simulink model "highspeed_iobuf_ex"  (Simulink 7.1)
settings: Solver=ode45  StartTime=0.0  StopTime=1000  RelTol=1e-3
libraries: xbsIndex_r4 x32, xbsCopyrightNotice_r4 x1
settings Model: Creator=alexc  LastModifiedBy=juttu
settings DataIOCC: SignalLoggingName=sigsOut
settings DebuggingCC: SaveWithParameterizedLinksMsg=none  SignalResolutionControl=TryResolveAllWithWarning  SolverPrmCheckMsg=none  MultiTaskDSMMsg=warning  MultiTaskCondExecSysMsg=none  StrictBusMsg=None
settings HardwareCC: TargetUnknown=on
settings RTWCC: IncludeERTFirstTime=on
settings GRTTargetCC: TargetFcnLib=ansi_tfl_tmw.mat

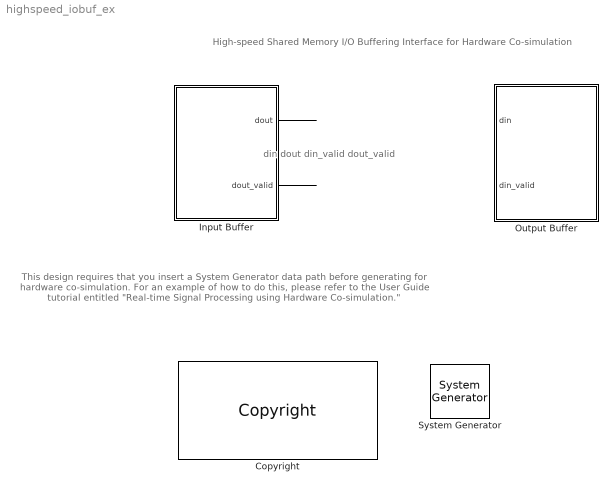
== system highspeed_iobuf_ex ==
  note: din                     dout
      |
      |
      |
      |
      | din_valid   dout_valid
  note: High-speed Shared Memory I/O Buffering Interface
      | for Hardware Co-simulation
  note: This design requires that you insert a System Generator
      | data path before generating for hardware co-simulation.
      | For an example of how to do this, please refer to the User
      | Guide tutorial entitled "Real-time Signal Processing using
      | Hardware Co-simulation."
  " System Generator" : xbsIndex_r4/ System Generator  Tag=genX  SystemSampleTime=-1  xilinxfamily=virtex4  part=xc4vsx35  speed=-10  package=ff668  synthesis_tool=XST  clock_wrapper=Clock Enables  directory=./netlist  testbench=off  simulink_period=1  sysclk_period=25  dcm_input_clock_period=100  incr_netlist=off  trim_vbits=Everywhere in SubSystem  dbl_ovrd=According to Block Masks  core_generation=According to Block Masks  run_coregen=off  deprecated_control=off  eval_field=0  block_type=sysgen
      settings: block_version=11.1
  Copyright : xbsCopyrightNotice_r4/Copyright  copyrighttext="Copyright (c) 2009  by  Xilinx, Inc. All rights reserved.<br><br>This file contains proprietary, confidential information of Xilinx, Inc., is distributed under licensefrom Xilinx, Inc., and may be used, copied and/or disclosed only pursuant to the terms of a valid licenseagreement with Xilinx, Inc. Xilinx hereby grants you a license to use this file solely for design,simulation, implementation and creation of design files limited to Xilinx devices or technologies. Use with non-Xilinx devices or technologies is expressly prohibited and immediately terminates your license unless covered by a separate agreement.<br><br>Xilinx is providing this design, code, or information \"as-is\" solely for use in developing programs and solutions for Xilinx devices, with no obligation on the part of Xilinx to provide support. By providingthis design, code, or information as one possible implementation of this feature, application or standard,Xilinx is making no representation that this implementation is free from any claims of infringement. Youare responsible for obtaining any rights you may require for your implementation. Xilinx expressly disclaimsany warranty whatsoever with respect to the adequacy of the implementation, including but not limited to anywarranties or representations that this implementation is free from claims of infringement, implied warrantiesof merchantability or fitness for a particular purpose.<br><br>Xilinx products are not intended for use in life support appliances, devices, or systems. Use in such applications is expressly prohibited.<br><br>Any modifications that are made to the Source Code are done at the user's sole risk and will be unsupported.<br><br>This copyright and support notice must be retained as part of this text at all times. (c) Copyright 1995-2009 Xilinx, Inc. All rights reserved."  block_type=copyright
      settings: block_version=11.1
  Input Buffer : Subsystem  mask{smName='Foo', smDepth=128*128, smWidth=8}
      mask prompts: smName "Shared Memory Name"; smDepth "Shared Memory Depth"; smWidth "Shared Memory Width"
  Output Buffer : Subsystem  mask{smName='Bar', smDepth=128*128}
      mask prompts: smName "Shared Memory Name"; smDepth "Shared Memory Depth"
  wires:
  Input Buffer/1(dout) -> ?
  Input Buffer/2(dout_valid) -> ?
  ? -> Output Buffer/1(din)
  ? -> Output Buffer/2(din_valid)

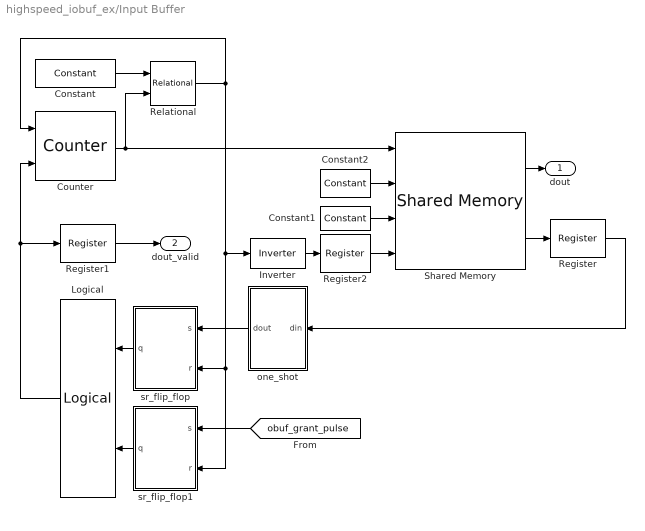
== system highspeed_iobuf_ex/Input Buffer ==
  Constant : xbsIndex_r4/Constant  arith_type=Unsigned  const=smDepth-1  n_bits=ceil(log2(smDepth))  bin_pt=0  explicit_period=on  period=1  equ=P=C  opselect=C  inp2=PCIN>>17  opr=+  inp1=P  carry=CIN  dbl_ovrd=off  block_type=constant
      settings: block_version=VER_STRING_GOES_HERE
  Constant1 : xbsIndex_r4/Constant  arith_type=Boolean  const=0  n_bits=1  bin_pt=0  explicit_period=off  period=1  equ=P=C  opselect=C  inp2=PCIN>>17  opr=+  inp1=P  carry=CIN  dbl_ovrd=off  block_type=constant
      settings: block_version=VER_STRING_GOES_HERE
  Constant2 : xbsIndex_r4/Constant  arith_type=Unsigned  const=0  n_bits=smWidth  bin_pt=0  explicit_period=off  period=1  equ=P=C  opselect=C  inp2=PCIN>>17  opr=+  inp1=P  carry=CIN  dbl_ovrd=off  block_type=constant
      settings: block_version=VER_STRING_GOES_HERE
  Counter : xbsIndex_r4/Counter  cnt_type=Free Running  cnt_to=Inf  operation=Up  start_count=0  cnt_by_val=1  arith_type=Unsigned  n_bits=ceil(log2(smDepth))  bin_pt=0  load_pin=off  rst=on  en=on  dbl_ovrd=off  explicit_period=on  period=1  use_behavioral_HDL=off  use_rpm=off  block_type=counter
      settings: infoedit="Configurable up, down and up/down counter.<P><P>Hardware notes: Free running counters are the least expensive in hardware.  A count limited counter is implemented by combining a counter with a comparator."  xl_area=[0, 0, 0, 0, 0, 0, 0]  block_version=VER_STRING_GOES_HERE
  Inverter : xbsIndex_r4/Inverter  en=off  latency=0  dbl_ovrd=off  block_type=inv
      settings: xl_area=[0, 0, 0, 0, 0, 0, 0]  block_version=VER_STRING_GOES_HERE
  Logical : xbsIndex_r4/Logical  Orientation=left  logical_function=AND  inputs=2  en=off  latency=0  precision=Full  arith_type=Unsigned  n_bits=8  bin_pt=2  align_bp=on  dbl_ovrd=off  block_type=logical
      settings: xl_area=[0, 0, 0, 0, 0, 0, 0]  block_version=VER_STRING_GOES_HERE
  Register : xbsIndex_r4/Register  init=0  rst=off  en=off  dbl_ovrd=off  block_type=register
      settings: xl_area=[0, 0, 0, 0, 0, 0, 0]  block_version=VER_STRING_GOES_HERE
  Register1 : xbsIndex_r4/Register  init=0  rst=off  en=off  dbl_ovrd=off  block_type=register
      settings: xl_area=[0, 0, 0, 0, 0, 0, 0]  block_version=VER_STRING_GOES_HERE
  Register2 : xbsIndex_r4/Register  init=0  rst=off  en=off  dbl_ovrd=off  block_type=register
      settings: xl_area=[0, 0, 0, 0, 0, 0, 0]  block_version=VER_STRING_GOES_HERE
  Relational : xbsIndex_r4/Relational  mode=a=b  en=off  latency=0  dbl_ovrd=off  block_type=relational
      settings: xl_area=[0, 0, 0, 0, 0, 0, 0]  block_version=VER_STRING_GOES_HERE
  Shared Memory : xbsIndex_r4/Shared Memory  shared_memory_name=smName  depth=smDepth  ownership=Locally Owned and Initialized  initVector=0:255  mutex=Lockable  mode=Read and Write  write_mode=Read After Write  time_out=0  explicit_data_type=off  arith_type=Unsigned  n_bits=0  bin_pt=0  implementation=Block RAM  use_rpm=off  block_type=shmem
      settings: AttributesFormatString=<< %<shared_memory_name> >>  xl_area=[0, 0, 0, 0, 0, 0, 0]  block_version=VER_STRING_GOES_HERE
  one_shot : Subsystem  Orientation=left
  sr_flip_flop : Subsystem  Orientation=left
  sr_flip_flop1 : Subsystem  Orientation=left
  dout : Outport  OutDataType=sfix(16)  OutScaling=2^0
  dout_valid : Outport  Port=2  OutDataType=sfix(16)  OutScaling=2^0
  wires:
  Shared Memory/2 -> Register/1
  Counter/1 -> Shared Memory/1, Relational/2
  Constant/1 -> Relational/1
  Relational/1 -> Inverter/1, sr_flip_flop/2(r), sr_flip_flop1/2(r), Counter/1
  Inverter/1 -> Register2/1
  Register2/1 -> Shared Memory/4
  Constant1/1 -> Shared Memory/3
  Constant2/1 -> Shared Memory/2
  [obuf_grant_pulse] -> sr_flip_flop1/1(s)
  one_shot/1(dout) -> sr_flip_flop/1(s)
  sr_flip_flop1/1(q) -> Logical/2
  sr_flip_flop/1(q) -> Logical/1
  Logical/1 -> Counter/2, Register1/1
  Register/1 -> one_shot/1(din)
  Register1/1 -> dout_valid/1
  Shared Memory/1 -> dout/1

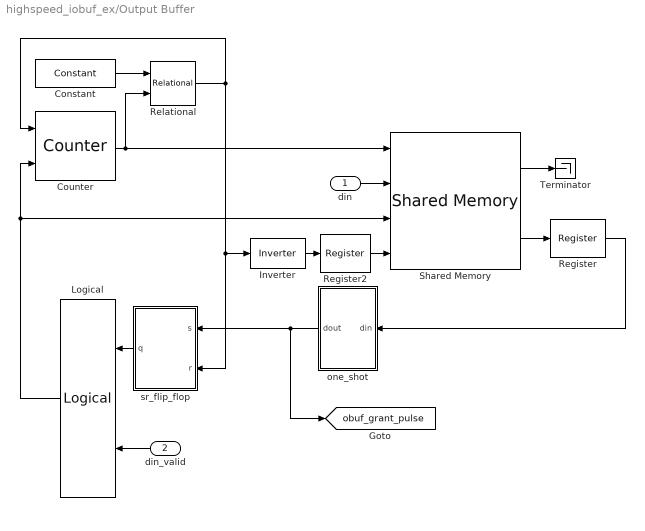
== system highspeed_iobuf_ex/Output Buffer ==
  din : Inport  OutDataType=sfix(16)  OutScaling=2^0
  din_valid : Inport  Orientation=left  Port=2  OutDataType=sfix(16)  OutScaling=2^0
  Constant : xbsIndex_r4/Constant  arith_type=Unsigned  const=smDepth-1  n_bits=ceil(log2(smDepth))  bin_pt=0  explicit_period=on  period=1  equ=P=C  opselect=C  inp2=PCIN>>17  opr=+  inp1=P  carry=CIN  dbl_ovrd=off  block_type=constant
      settings: block_version=VER_STRING_GOES_HERE
  Counter : xbsIndex_r4/Counter  cnt_type=Free Running  cnt_to=Inf  operation=Up  start_count=0  cnt_by_val=1  arith_type=Unsigned  n_bits=ceil(log2(smDepth))  bin_pt=0  load_pin=off  rst=on  en=on  dbl_ovrd=off  explicit_period=on  period=1  use_behavioral_HDL=off  use_rpm=off  block_type=counter
      settings: infoedit="Configurable up, down and up/down counter.<P><P>Hardware notes: Free running counters are the least expensive in hardware.  A count limited counter is implemented by combining a counter with a comparator."  xl_area=[0, 0, 0, 0, 0, 0, 0]  block_version=VER_STRING_GOES_HERE
  Inverter : xbsIndex_r4/Inverter  en=off  latency=0  dbl_ovrd=off  block_type=inv
      settings: xl_area=[0, 0, 0, 0, 0, 0, 0]  block_version=VER_STRING_GOES_HERE
  Logical : xbsIndex_r4/Logical  Orientation=left  logical_function=AND  inputs=2  en=off  latency=0  precision=Full  arith_type=Unsigned  n_bits=8  bin_pt=2  align_bp=on  dbl_ovrd=off  block_type=logical
      settings: xl_area=[0, 0, 0, 0, 0, 0, 0]  block_version=VER_STRING_GOES_HERE
  Register : xbsIndex_r4/Register  init=0  rst=off  en=off  dbl_ovrd=off  block_type=register
      settings: xl_area=[0, 0, 0, 0, 0, 0, 0]  block_version=VER_STRING_GOES_HERE
  Register2 : xbsIndex_r4/Register  init=0  rst=off  en=off  dbl_ovrd=off  block_type=register
      settings: xl_area=[0, 0, 0, 0, 0, 0, 0]  block_version=VER_STRING_GOES_HERE
  Relational : xbsIndex_r4/Relational  mode=a=b  en=off  latency=0  dbl_ovrd=off  block_type=relational
      settings: xl_area=[0, 0, 0, 0, 0, 0, 0]  block_version=VER_STRING_GOES_HERE
  Shared Memory : xbsIndex_r4/Shared Memory  shared_memory_name=smName  depth=smDepth  ownership=Locally Owned and Initialized  initVector=0  mutex=Lockable  mode=Read and Write  write_mode=Read After Write  time_out=0  explicit_data_type=off  arith_type=Unsigned  n_bits=0  bin_pt=0  implementation=Block RAM  use_rpm=off  block_type=shmem
      settings: AttributesFormatString=<< %<shared_memory_name> >>  xl_area=[0, 0, 0, 0, 0, 0, 0]  block_version=VER_STRING_GOES_HERE
  Terminator : Terminator
  one_shot : Subsystem  Orientation=left
  sr_flip_flop : Subsystem  Orientation=left
  tag scope: obuf_grant_pulse=global
  wires:
  Shared Memory/1 -> Terminator/1
  Register/1 -> one_shot/1(din)
  Logical/1 -> Counter/2, Shared Memory/3
  sr_flip_flop/1(q) -> Logical/1
  one_shot/1(dout) -> sr_flip_flop/1(s), [obuf_grant_pulse]
  Register2/1 -> Shared Memory/4
  Inverter/1 -> Register2/1
  Relational/1 -> Counter/1, Inverter/1, sr_flip_flop/2(r)
  Constant/1 -> Relational/1
  Counter/1 -> Relational/2, Shared Memory/1
  Shared Memory/2 -> Register/1
  din_valid/1 -> Logical/2
  din/1 -> Shared Memory/2

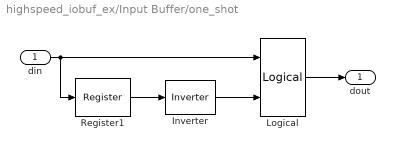
== system highspeed_iobuf_ex/Input Buffer/one_shot ==
  din : Inport  OutDataType=sfix(16)  OutScaling=2^0
  Inverter : xbsIndex_r4/Inverter  en=off  latency=0  dbl_ovrd=off  block_type=inv
      settings: xl_area=[0, 0, 0, 0, 0, 0, 0]  block_version=VER_STRING_GOES_HERE
  Logical : xbsIndex_r4/Logical  logical_function=AND  inputs=2  en=off  latency=0  precision=Full  arith_type=Unsigned  n_bits=8  bin_pt=2  align_bp=on  dbl_ovrd=off  block_type=logical
      settings: xl_area=[0, 0, 0, 0, 0, 0, 0]  block_version=VER_STRING_GOES_HERE
  Register1 : xbsIndex_r4/Register  init=0  rst=off  en=off  dbl_ovrd=off  block_type=register
      settings: xl_area=[0, 0, 0, 0, 0, 0, 0]  block_version=VER_STRING_GOES_HERE
  dout : Outport  OutDataType=sfix(16)  OutScaling=2^0
  wires:
  din/1 -> Register1/1, Logical/1
  Register1/1 -> Inverter/1
  Inverter/1 -> Logical/2
  Logical/1 -> dout/1

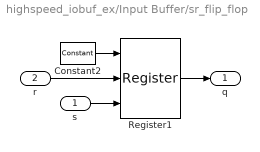
== system highspeed_iobuf_ex/Input Buffer/sr_flip_flop ==
  s : Inport  OutDataType=sfix(16)  OutScaling=2^0
  r : Inport  Port=2  OutDataType=sfix(16)  OutScaling=2^0
  Constant2 : xbsIndex_r4/Constant  arith_type=Boolean  const=1  n_bits=1  bin_pt=0  explicit_period=off  period=1  equ=P=C  opselect=C  inp2=PCIN>>17  opr=+  inp1=P  carry=CIN  dbl_ovrd=off  block_type=constant
      settings: block_version=VER_STRING_GOES_HERE
  Register1 : xbsIndex_r4/Register  init=0  rst=on  en=on  dbl_ovrd=off  block_type=register
      settings: xl_area=[0, 0, 0, 0, 0, 0, 0]  block_version=VER_STRING_GOES_HERE
  q : Outport  OutDataType=sfix(16)  OutScaling=2^0
  wires:
  Register1/1 -> q/1
  Constant2/1 -> Register1/1
  r/1 -> Register1/2
  s/1 -> Register1/3

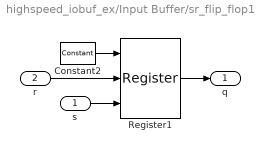
== system highspeed_iobuf_ex/Input Buffer/sr_flip_flop1 ==
  s : Inport  OutDataType=sfix(16)  OutScaling=2^0
  r : Inport  Port=2  OutDataType=sfix(16)  OutScaling=2^0
  Constant2 : xbsIndex_r4/Constant  arith_type=Boolean  const=1  n_bits=1  bin_pt=0  explicit_period=off  period=1  equ=P=C  opselect=C  inp2=PCIN>>17  opr=+  inp1=P  carry=CIN  dbl_ovrd=off  block_type=constant
      settings: block_version=VER_STRING_GOES_HERE
  Register1 : xbsIndex_r4/Register  init=0  rst=on  en=on  dbl_ovrd=off  block_type=register
      settings: xl_area=[0, 0, 0, 0, 0, 0, 0]  block_version=VER_STRING_GOES_HERE
  q : Outport  OutDataType=sfix(16)  OutScaling=2^0
  wires:
  s/1 -> Register1/3
  r/1 -> Register1/2
  Constant2/1 -> Register1/1
  Register1/1 -> q/1

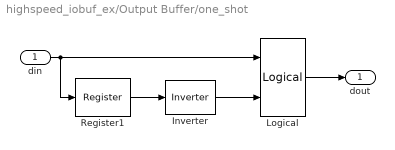
== system highspeed_iobuf_ex/Output Buffer/one_shot ==
  din : Inport  OutDataType=sfix(16)  OutScaling=2^0
  Inverter : xbsIndex_r4/Inverter  en=off  latency=0  dbl_ovrd=off  block_type=inv
      settings: xl_area=[0, 0, 0, 0, 0, 0, 0]  block_version=VER_STRING_GOES_HERE
  Logical : xbsIndex_r4/Logical  logical_function=AND  inputs=2  en=off  latency=0  precision=Full  arith_type=Unsigned  n_bits=8  bin_pt=2  align_bp=on  dbl_ovrd=off  block_type=logical
      settings: xl_area=[0, 0, 0, 0, 0, 0, 0]  block_version=VER_STRING_GOES_HERE
  Register1 : xbsIndex_r4/Register  init=0  rst=off  en=off  dbl_ovrd=off  block_type=register
      settings: xl_area=[0, 0, 0, 0, 0, 0, 0]  block_version=VER_STRING_GOES_HERE
  dout : Outport  OutDataType=sfix(16)  OutScaling=2^0
  wires:
  Logical/1 -> dout/1
  Inverter/1 -> Logical/2
  Register1/1 -> Inverter/1
  din/1 -> Logical/1, Register1/1

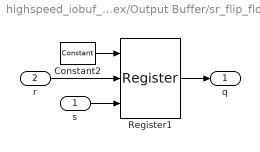
== system highspeed_iobuf_ex/Output Buffer/sr_flip_flop ==
  s : Inport  OutDataType=sfix(16)  OutScaling=2^0
  r : Inport  Port=2  OutDataType=sfix(16)  OutScaling=2^0
  Constant2 : xbsIndex_r4/Constant  arith_type=Boolean  const=1  n_bits=1  bin_pt=0  explicit_period=off  period=1  equ=P=C  opselect=C  inp2=PCIN>>17  opr=+  inp1=P  carry=CIN  dbl_ovrd=off  block_type=constant
      settings: block_version=VER_STRING_GOES_HERE
  Register1 : xbsIndex_r4/Register  init=0  rst=on  en=on  dbl_ovrd=off  block_type=register
      settings: xl_area=[0, 0, 0, 0, 0, 0, 0]  block_version=VER_STRING_GOES_HERE
  q : Outport  OutDataType=sfix(16)  OutScaling=2^0
  wires:
  s/1 -> Register1/3
  r/1 -> Register1/2
  Constant2/1 -> Register1/1
  Register1/1 -> q/1
